simulink model "Question_8_simulation"  (R2020a)
settings: Solver=VariableStepAuto  StartTime=0.0  StopTime=10.0  RelTol=1e-3
settings Model: Creator=Noémie  LastModifiedBy=Noémie

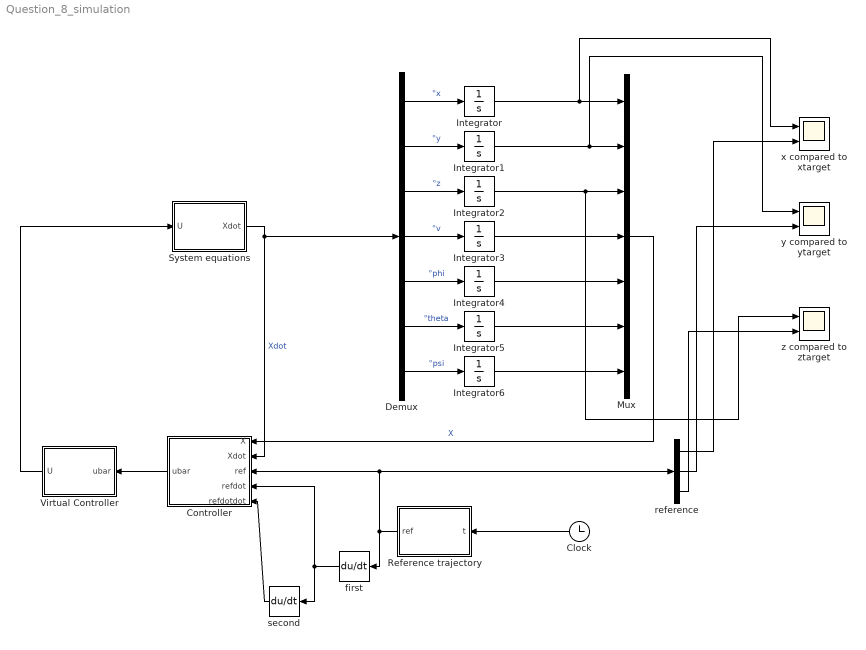
== system Question_8_simulation ==
  Clock : Clock
  Controller : MATLAB Function  TreatAsAtomicUnit=on
  Demux : Demux  Outputs=7
  Integrator{,1..2,4..6} (6 alike) : Integrator
  Integrator3 : Integrator  InitialCondition=1
  Mux : Mux  Inputs=7
  Reference trajectory : MATLAB Function  TreatAsAtomicUnit=on
  System equations : MATLAB Function  TreatAsAtomicUnit=on
  Virtual Controller : MATLAB Function  TreatAsAtomicUnit=on
  first : Derivative
  reference : Demux  Outputs=3
  second : Derivative
  x compared to xtarget : Scope  NumInputPorts=2
  y compared to ytarget : Scope  NumInputPorts=2
  z compared to ztarget : Scope  NumInputPorts=2
  wires:
  Controller/1(ubar) -> Virtual Controller/1(ubar)
  Clock/1 -> Reference trajectory/1(t)
  Reference trajectory/1(ref) -> first/1, reference/1, Controller/3(ref)
  first/1 -> second/1, Controller/4(refdot)
  second/1 -> Controller/5(refdotdot)
  Virtual Controller/1(U) -> System equations/1(U)
  Integrator/1 -> x compared to xtarget/1, Mux/1
  Demux/6 -> Integrator5/1  "°theta"
  Integrator5/1 -> Mux/6
  Demux/5 -> Integrator4/1  "°phi"
  Integrator6/1 -> Mux/7
  Demux/4 -> Integrator3/1  "°v"
  Integrator1/1 -> y compared to ytarget/1, Mux/2
  Demux/2 -> Integrator1/1  "°y"
  Integrator2/1 -> z compared to ztarget/1, Mux/3
  Demux/7 -> Integrator6/1  "°psi"
  Integrator3/1 -> Mux/4
  Demux/3 -> Integrator2/1  "°z"
  Demux/1 -> Integrator/1  "°x"
  Integrator4/1 -> Mux/5
  System equations/1(Xdot) -> Demux/1, Controller/2(Xdot)  "Xdot"
  Mux/1 -> Controller/1(X)  "X"
  reference/1 -> x compared to xtarget/2
  reference/2 -> y compared to ytarget/2
  reference/3 -> z compared to ztarget/2

== matlab function Question_8_simulation/Controller ==
  data: X input; Xdot input; ref input; ubar output; refdot input; refdotdot input
function ubar = fcn(X, Xdot, ref, refdot, refdotdot)

ubar1 = (ref(1) - X(1)) + 2 * (refdot(1) - Xdot(1)) + refdotdot(1);
ubar2 = (ref(2) - X(2)) + 2 * (refdot(2) - Xdot(2)) + refdotdot(2);
ubar3 = (ref(3) - X(3)) + 2 * (refdot(3) - Xdot(3)) + refdotdot(3);

ubar = [ubar1, ubar2, ubar3];

== matlab function Question_8_simulation/System equations ==
  data: U input; Xdot output
function Xdot = fcn(U)

u_1 = U(1);
u_2 = U(2);
u_3 = U(3);

X_dot = [v*cos(theta)*cos(psi), v*cos(theta)*sin(psi), -v*sin(theta)];
v_dot = u_1;
phi_dot = -0.1*sin(phi)*cos(theta)+v*tan(theta)*(u_2*sin(phi)+u_3*cos(phi));
theta_dot = v*u_2*cos(phi)-v*u_3*sin(phi);
psi_dot = v*u_2*(sin(phi)/cos(theta)) + v*u_3*(cos(phi)/cos(theta));

Xdot = [X_dot, v_dot, phi_dot, theta_dot, psi_dot];

== matlab function Question_8_simulation/Virtual Controller ==
  data: ubar input; U output
function U = fcn(ubar)

Ainverse = [cos(psi)*cos(theta), cos(theta)*sin(psi), -sin(theta);
            -(sin(phi)*sin(psi) + cos(phi)*cos(psi)*sin(theta))/v^2, (cos(psi)*sin(phi) - cos(phi)*sin(psi)*sin(theta))/v^2, -(cos(phi)*cos(theta))/v^2;
            -(cos(phi)*sin(psi) - cos(psi)*sin(phi)*sin(theta))/v^2, (cos(phi)*cos(psi) + sin(phi)*sin(psi)*sin(theta))/v^2, (cos(theta)*sin(phi))/v^2];


U = Ainverse * ubar;

== matlab function Question_8_simulation/Reference trajectory ==
  data: t input; ref output
function ref = fcn(t)

xtarget = 20 * sin( 1 * t ) + 20 * sin( 6 * t );

ytarget = 20 * cos( 1 * t ) + 20 * cos( 6 * t );

ztarget = 20 * sin( 0.2 * t );

ref = [xtarget, ytarget, ztarget];
